simulink model "Q4_2"  (R2021a)
settings: Solver=FixedStepAuto  StartTime=0.0  StopTime=60  FixedStep=0.001  RelTol=1e-3
settings Model: Creator=M.M  LastModifiedBy=M.M

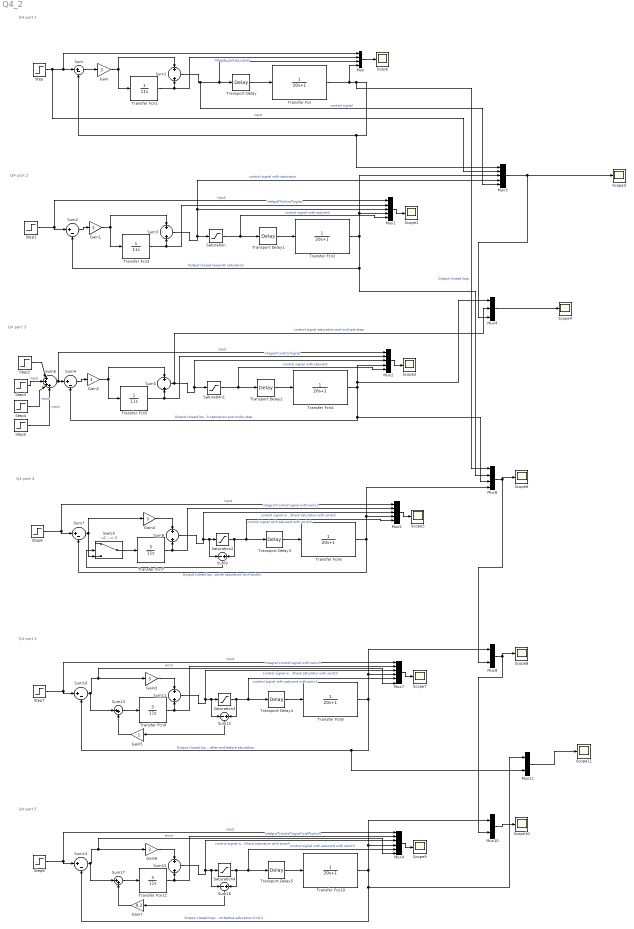
== system Q4_2 ==
  note: Q4 part 1
  note: Q4 part 2
  note: Q4 part 3
  note: Q4 part 4
  note: Q4 part 5
  note: Q4 part 5
  Gain{,1..4,6} (6 alike) : Gain  Gain=3
  Gain5 : Gain
  Gain7 : Gain  Gain=0.2
  Mux : Mux
  Mux{1..3,5} (4 alike) : Mux  Inputs=5
  Mux10 : Mux  Inputs=2
  Mux11 : Mux  Inputs=2
  Mux4 : Mux  Inputs=3
  Mux6 : Mux
  Mux7 : Mux  Inputs=6
  Mux8 : Mux  Inputs=2
  Mux9 : Mux  Inputs=6
  Saturation{,1..4} (5 alike) : Saturate  UpperLimit=2  LowerLimit=-2
  Scope{,1..11} (12 alike) : Scope
  Step{,1,6..8} (5 alike) : Step  Time=0  SampleTime=0
  Step2 : Step  Time=0  After=0.25  SampleTime=0
  Step3 : Step  Time=7  After=0.25  SampleTime=0
  Step4 : Step  Time=14  After=0.25  SampleTime=0
  Step5 : Step  Time=21  After=0.25  SampleTime=0
  Sum{,2,4,7,10,14} (6 alike) : Sum  Inputs=|+-
  Sum{1,3,5,8,11,15} (6 alike) : Sum  Inputs=+|||+
  Sum12 : Sum  Inputs=-+
  Sum13 : Sum  Inputs=|++
  Sum16 : Sum  Inputs=-+
  Sum17 : Sum  Inputs=|++
  Sum6 : Sum  Inputs=|++++
  Sum9 : Sum  Inputs=-+
  Switch : Switch  Criteria=u2 ~= 0
  Transfer Fcn{,2,4,6,8,10} (6 alike) : TransferFcn  Denominator=[20 1]
  Transfer Fcn1 : TransferFcn  Denominator=[11 0]
  Transfer Fcn11 : TransferFcn  Numerator=[3]  Denominator=[11 0]
  Transfer Fcn3 : TransferFcn  Denominator=[11 0]
  Transfer Fcn5 : TransferFcn  Denominator=[11 0]
  Transfer Fcn7 : TransferFcn  Numerator=[3]  Denominator=[11 0]
  Transfer Fcn9 : TransferFcn  Numerator=[3]  Denominator=[11 0]
  Transport Delay{,1..5} (6 alike) : TransportDelay  DelayTime=4
  wires:
  Transfer Fcn/1 -> Mux/4, Mux6/1, Mux3/1, Sum/2  "Output closed loop"
  Transport Delay/1 -> Transfer Fcn/1
  Step/1 -> Mux3/2, Mux/1, Sum/1  "input"
  Sum/1 -> Gain/1
  Sum1/1 -> Mux3/5, Mux/3, Transport Delay/1  "control signal"
  Gain/1 -> Transfer Fcn1/1, Sum1/1
  Transfer Fcn1/1 -> Mux/2, Sum1/2  "integral control signal"
  Mux/1 -> Scope/1
  Transfer Fcn3/1 -> Mux1/2, Sum3/2  "integral control signal"
  Sum3/1 -> Mux3/4, Mux1/3, Saturation/1  "control signal with saturatun"
  Sum2/1 -> Gain1/1
  Step1/1 -> Mux1/1, Sum2/1  "input"
  Transport Delay1/1 -> Transfer Fcn2/1
  Mux1/1 -> Scope1/1
  Gain1/1 -> Transfer Fcn3/1, Sum3/1
  Transfer Fcn2/1 -> Mux6/2, Sum2/2, Mux3/3, Mux1/4  "Output closed loopwith saturation"
  Saturation/1 -> Mux1/5, Transport Delay1/1  "control signal with saturant"
  Gain2/1 -> Transfer Fcn5/1, Sum5/1
  Sum5/1 -> Mux4/2, Mux2/3, Saturation1/1  "control signal satyration and multiple step"
  Sum4/1 -> Gain2/1
  Transfer Fcn4/1 -> Mux4/1, Mux2/4, Mux6/3, Sum4/2  "Output closed loop with saturation and multy step"
  Transfer Fcn5/1 -> Mux2/2, Sum5/2  "integral control signal"
  Saturation1/1 -> Mux2/5, Transport Delay2/1  "control signal with saturant"
  Mux2/1 -> Scope2/1
  Transport Delay2/1 -> Transfer Fcn4/1
  Sum6/1 -> Mux2/1, Sum4/1  "input"
  Step2/1 -> Sum6/1
  Step3/1 -> Sum6/2  "input"
  Step4/1 -> Sum6/3  "input"
  Step5/1 -> Sum6/4  "input"
  Mux3/1 -> Mux4/3, Scope3/1
  Mux4/1 -> Scope4/1
  Sum8/1 -> Mux5/3, Sum9/1, Saturation2/1  "control signal without saturatun with switch"
  Sum7/1 -> Switch/3, Gain4/1
  Transfer Fcn6/1 -> Mux6/4, Mux5/4, Sum7/2  "Output closed loopwith saturation with switch"
  Step6/1 -> Mux5/1, Sum7/1  "input"
  Transport Delay3/1 -> Transfer Fcn6/1
  Saturation2/1 -> Sum9/2, Mux5/5, Transport Delay3/1  "control signal with saturant with switch"
  Transfer Fcn7/1 -> Mux5/2, Sum8/2  "integral control signal with switch"
  Mux5/1 -> Scope5/1
  Gain4/1 -> Sum8/1
  Switch/1 -> Transfer Fcn7/1
  Sum9/1 -> Switch/2
  Mux6/1 -> Mux8/2, Scope6/1
  Sum13/1 -> Transfer Fcn9/1
  Mux7/1 -> Scope7/1
  Step7/1 -> Mux7/1, Sum10/1  "input"
  Sum11/1 -> Mux7/3, Sum12/1, Saturation3/1  "control signal without saturatun with switch"
  Transfer Fcn9/1 -> Mux7/2, Sum11/2  "integral control signal with switch"
  Gain3/1 -> Sum11/1
  Sum10/1 -> Sum13/1, Mux7/6, Gain3/1  "error"
  Saturation3/1 -> Sum12/2, Mux7/5, Transport Delay4/1  "control signal with saturant with switch"
  Transfer Fcn8/1 -> Mux8/1, Mux7/4, Mux11/2, Sum10/2  "Output closed loopwith saturation with signal of error of after and before saturation"
  Transport Delay4/1 -> Transfer Fcn8/1
  Sum12/1 -> Gain5/1
  Gain5/1 -> Sum13/2
  Transport Delay5/1 -> Transfer Fcn10/1
  Mux8/1 -> Mux10/2, Scope8/1
  Gain7/1 -> Sum17/2
  Saturation4/1 -> Sum16/2, Mux9/5, Transport Delay5/1  "control signal with saturant with switch"
  Sum16/1 -> Gain7/1
  Sum14/1 -> Sum17/1, Mux9/6, Gain6/1  "error"
  Gain6/1 -> Sum15/1
  Transfer Fcn11/1 -> Mux9/2, Sum15/2  "integral control signal with switch"
  Sum17/1 -> Transfer Fcn11/1
  Transfer Fcn10/1 -> Mux10/1, Mux9/4, Mux11/1, Sum14/2  "Output closed loopwith saturation with signal of error of after and before saturation ti=0.2"
  Sum15/1 -> Mux9/3, Sum16/1, Saturation4/1  "control signal without saturatun with switch"
  Step8/1 -> Mux9/1, Sum14/1  "input"
  Mux9/1 -> Scope9/1
  Mux10/1 -> Scope10/1
  Mux11/1 -> Scope11/1
